simulink model "rigid_body_model"  (R2025b)
settings: Solver=ode4  StartTime=0  StopTime=10.0  FixedStep=0.001  RelTol=1e-3  EnableMultiTasking=on
undefined symbols (not defined in the file or in its folder): DiscIntNeverNeededParam
libraries: vrlib x2, aerolibutil x1
settings Model: DataDictionary=pid.sldd  EnableAccessToBaseWorkspace=off  ModifiedByFormat=The MathWorks Inc.  Creator=The MathWorks, Inc.  LastModifiedBy=The MathWorks Inc.
settings SolverCC: AlgebraicLoopSolver=TrustRegion
settings DataIOCC: ReturnWorkspaceOutputs=off
settings OptimizationCC: BlockReduction=off  DefaultParameterBehavior=Inlined  InlineInvariantSignals=on  BufferReuse=off  PassReuseOutputArgsAs=Individual arguments  ExpressionDepthLimit=2147483647.0  ZeroExternalMemoryAtStartup=off  ZeroInternalMemoryAtStartup=off  EfficientFloat2IntCast=on  LifeSpan=1  EfficientTunableParamExpr=on
settings DebuggingCC: AlgebraicLoopMsg=none  FcnCallInpInsideContextMsg=warning  UniqueDataStoreMsg=error  AssertControl=DisableAll  AllowSymbolicDim=off  StateNameClashWarn=warning  StrictBusMsg=ErrorOnBusTreatedAsVector  SFUnexpectedBacktrackingDiag=warning  SFNoUnconditionalDefaultTransitionDiag=warning  SFExecutionAtInitializationDiag=none  ArithmeticOperatorsInVariantConditions=warning
settings HardwareCC: ProdBitPerPointer=32.0  ProdBitPerSizeT=32.0  ProdBitPerPtrDiffT=32.0  ProdLargestAtomicFloat=None  ProdIntDivRoundTo=Undefined  ProdEndianess=Unspecified  ProdWordSize=32.0  ProdHWDeviceType=32-bit Generic
settings ModelReferenceCC: EnableRefExpFcnMdlSchedulingChecks=on  PropagateSignalLabelsOutOfModel=off
settings SFSimCC: SimUseLocalCustomCode=off  CustomCodeUndefinedFunction=UseInterfaceOnly
settings RTWCC: SystemTargetFile=ert.tlc  TemplateMakefile=ert_default_tmf  GenerateReport=on  RTWUseLocalCustomCode=off  IncludeHyperlinkInReport=on  GenerateTraceInfo=on  GenerateTraceReport=on  GenerateTraceReportSl=on  GenerateTraceReportSf=on  GenerateTraceReportEml=on  GenerateCodeMetricsReport=on  GPUComputeCapability=3.5  DLArmComputeVersion=19.05  Description=Embedded Coder
settings CodeAppCC: IgnoreCustomStorageClasses=off  IgnoreTestpoints=on  CustomSymbolStrType=$N$R$M  StateflowObjectComments=on  InternalIdentifier=Classic
settings ERTTargetCC: ERTCustomFileTemplate=example_file_process.tlc  ConvertIfToSwitch=off  SuppressUnreachableDefaultCases=off  DynamicArrayContainerType=coder::array  MultiwordLength=2048.0  GenerateSampleERTMain=on  SupportNonFinite=off  ParenthesesLevel=Maximum
settings ConfigComp: CovMetricSettings=dw  CovSaveCumulativeToWorkspaceVar=on  CovSaveSingleToWorkspaceVar=on  CovExternalEMLEnable=off  CovSFcnEnable=off

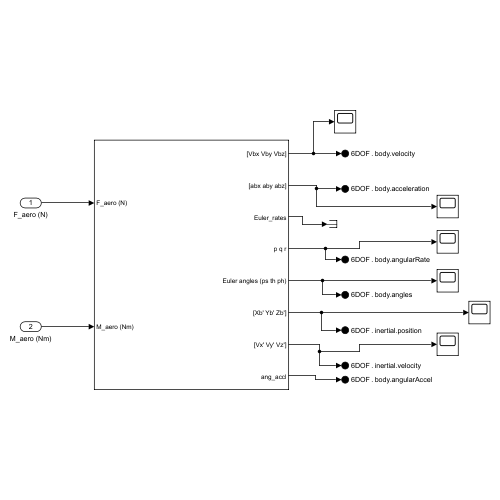
[thumbnail: Simulink's stored preview of the top-level diagram]
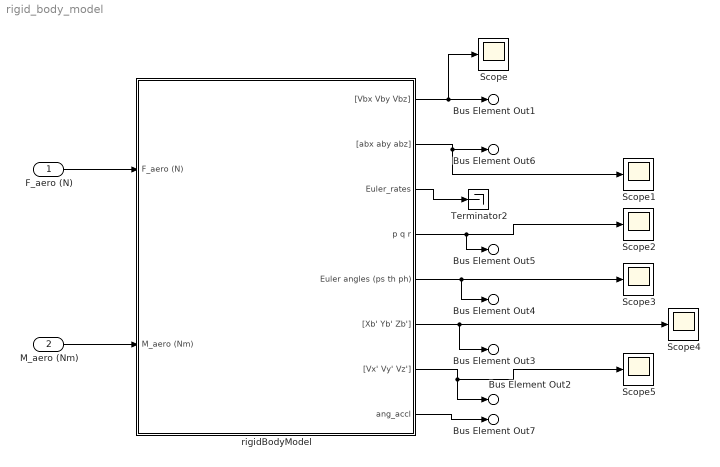
== system rigid_body_model ==
  F_aero (N) : Inport  PortDimensions=3
  M_aero (Nm) : Inport  Port=2  PortDimensions=3
  Scope{,1..5} (6 alike) : Scope
      Scope settings: ActiveDisplayYMinimum=-3.3667697972665165  ActiveDisplayYMaximum=3.6462998602310797
      Scope1 settings: ActiveDisplayYMinimum=-5.0415104437648826E+60  ActiveDisplayYMaximum=4.79275711289561E+60  DataLoggingVariableName=ScopeData2
      Scope2 settings: ActiveDisplayYMinimum=-3.6964469168621719  ActiveDisplayYMaximum=4.3336377029010054  DataLoggingVariableName=ScopeData3
      Scope3 settings: ActiveDisplayYMinimum=-0.15051515492555492  ActiveDisplayYMaximum=0.20760201896329444  DataLoggingVariableName=ScopeData4
      Scope4 settings: ActiveDisplayYMinimum=-0.00018500944845913292  ActiveDisplayYMaximum=0.0013947118751504368  DataLoggingVariableName=ScopeData5
      Scope5 settings: ActiveDisplayYMinimum=-74.102476128449538  ActiveDisplayYMaximum=562.81355446598127  DataLoggingVariableName=ScopeData6
  Terminator2 : Terminator
  rigidBodyModel : Subsystem
  Bus Element Out1 : Outport  PortName=6DOF  Element=body.velocity
  Bus Element Out4 : Outport  PortName=6DOF  Element=body.angles
  Bus Element Out6 : Outport  PortName=6DOF  Element=body.acceleration
  Bus Element Out5 : Outport  PortName=6DOF  Element=body.angularRate
  Bus Element Out7 : Outport  PortName=6DOF  Element=body.angularAccel
  Bus Element Out2 : Outport  PortName=6DOF  Element=inertial.velocity
  Bus Element Out3 : Outport  PortName=6DOF  Element=inertial.position
  wires:
  rigidBodyModel/1("[Vbx Vby Vbz]") -> Scope/1, Bus Element Out1/1
  rigidBodyModel/2("[abx aby abz]") -> Scope1/1, Bus Element Out6/1
  rigidBodyModel/3(Euler_rates) -> Terminator2/1
  rigidBodyModel/5(Euler angles (ps th ph)) -> Scope3/1, Bus Element Out4/1
  rigidBodyModel/4(p q r) -> Scope2/1, Bus Element Out5/1
  rigidBodyModel/7("[Vx' Vy' Vz']") -> Bus Element Out2/1, Scope5/1
  rigidBodyModel/6("[Xb' Yb' Zb']") -> Bus Element Out3/1, Scope4/1
  rigidBodyModel/8(ang_accl) -> Bus Element Out7/1
  M_aero (Nm)/1 -> rigidBodyModel/2(M_aero (Nm))
  F_aero (N)/1 -> rigidBodyModel/1(F_aero (N))

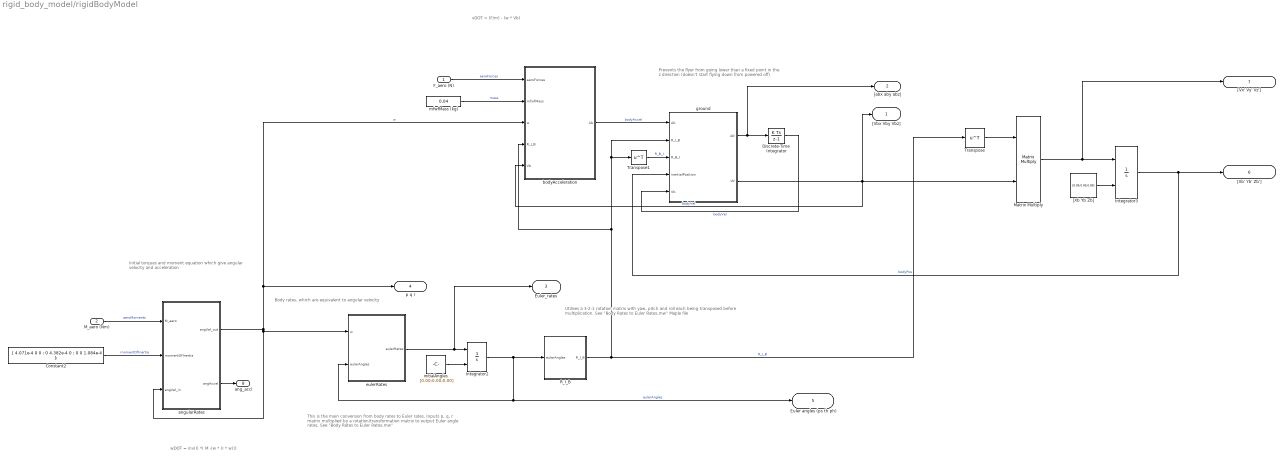
== system rigid_body_model/rigidBodyModel ==
  note: Utilises a 3-2-1 rotation matrix with yaw, pitch and roll each being transposed before multiplication. See "Body Rates to Euler Rates.mw" Maple file
  note: Prevents the flyer from going lower than a fixed point
      | in the z direction (doesn't start flying down from powered
      | off)
  note: Body rates, which are equivalent to angular velocity
  note: This is the main conversion from body rates to Euler rates.
      | Inputs p, q, r matrix multiplied by a rotation/transformation
      | matrix to output Euler angle rates. See "Body Rates to Euler Rates.mw"
  note: Initial torques and moment equation which give angular
      | velocity and acceleration
  note: wDOT = inv(I) *( M -(w * (I * w)))
  note: vDOT = (F/m) - (w * Vb)
  F_aero (N) : Inport
  M_aero (Nm) : Inport  Port=2
  Constant2 : Constant  Value=[ 4.071e-4 0 0 ; 0 4.382e-4 0 ; 0 0 1.084e-4 ];
  Discrete-Time Integrator : DiscreteIntegrator  SampleTime=-1  ICPrevOutput=DiscIntNeverNeededParam  ICPrevScaledInput=DiscIntNeverNeededParam
  Integrator2 : Integrator  InitialConditionSource=external
  Integrator3 : Integrator  InitialConditionSource=external  ShowStatePort=on
  Matrix Multiply : Product  Multiplication=Matrix(*)
  R_I_B : Subsystem
      mask Display: disp('R_I_B');
  Transpose : Math  Operator=transpose
  Transpose1 : Math  Operator=transpose
  "[Xb Yb Zb]" : Constant  Value=[0.00;0.00;0.00]
  angularRates : Subsystem
      mask Display: disp('Angular Rates');
  bodyAcceleration : Subsystem
      mask Display: disp('Body Acceleration');
  eulerRates : Subsystem
      mask Display: disp('Euler Rates');
  ground : Subsystem
      mask Display: disp('Ground');
  initialAngles : Constant  Value=[0.00;0.00;0.00]
  mfwfMass (kg) : Constant  Value=0.04
  "[Vbx Vby Vbz]" : Outport
  "[abx aby abz]" : Outport  Port=2
  Euler_rates : Outport  Port=3
  p q r : Outport  Port=4
  Euler angles (ps th ph) : Outport  Port=5
  "[Xb' Yb' Zb']" : Outport  Port=6
  "[Vx' Vy' Vz']" : Outport  Port=7
  ang_accl : Outport  Port=8
  wires:
  initialAngles/1 -> Integrator2/2
  M_aero (Nm)/1 -> angularRates/1(M_aero)  "aeroMoments"
  eulerRates/1(eulerRates) -> Integrator2/1, Euler_rates/1
  Transpose/1 -> Matrix Multiply/1
  "[Xb Yb Zb]"/1 -> Integrator3/2
  angularRates/1(angVel_out) -> angularRates/3(angVel_in), eulerRates/1(w), p q r/1, bodyAcceleration/3(w)  "w"
  Constant2/1 -> angularRates/2(momentOfInertia)  "momentOfInertia"
  Matrix Multiply/1 -> "[Vx' Vy' Vz']"/1, Integrator3/1
  ground/2(vb') -> "[Vbx Vby Vbz]"/1, Matrix Multiply/2, bodyAcceleration/5(Vb)  "bodyVel"
  Integrator3/1 -> "[Xb' Yb' Zb']"/1, ground/4(inertialPosition)  "bodyPos"
  Integrator2/1 -> Euler angles (ps th ph)/1, eulerRates/2(eulerAngles), R_I_B/1(eulerAngles)  "eulerAngles"
  R_I_B/1(R_I_B) -> bodyAcceleration/4(R_I_B), Transpose1/1, ground/2(R_I_B), Transpose/1  "R_I_B"
  angularRates/2(angAccel) -> ang_accl/1
  ground/1(Ab') -> "[abx aby abz]"/1, Discrete-Time Integrator/1
  Discrete-Time Integrator/1 -> ground/5(Vb)  "bodyVel"
  mfwfMass (kg)/1 -> bodyAcceleration/2(mfwfMass)  "mass"
  bodyAcceleration/1(Ab) -> ground/1(Ab)  "bodyAccel"
  Transpose1/1 -> ground/3(R_B_I)  "R_B_I"
  F_aero (N)/1 -> bodyAcceleration/1(aeroForces)  "aeroForces"

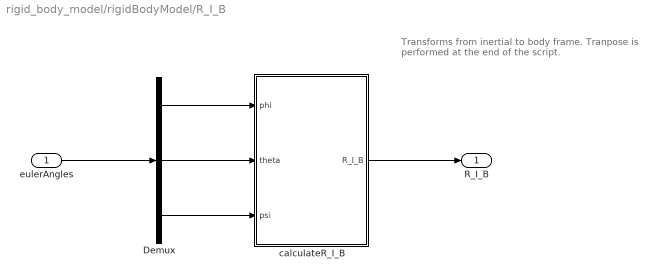
== system rigid_body_model/rigidBodyModel/R_I_B ==
  note: Transforms from inertial to body frame. Tranpose is
      | performed at the end of the script.
  eulerAngles : Inport
  Demux : Demux  Outputs=[1;1;1]
  calculateR_I_B : MATLAB Function  TreatAsAtomicUnit=on
  R_I_B : Outport
  wires:
  eulerAngles/1 -> Demux/1
  Demux/2 -> calculateR_I_B/2(theta)
  calculateR_I_B/1(R_I_B) -> R_I_B/1
  Demux/1 -> calculateR_I_B/1(phi)
  Demux/3 -> calculateR_I_B/3(psi)

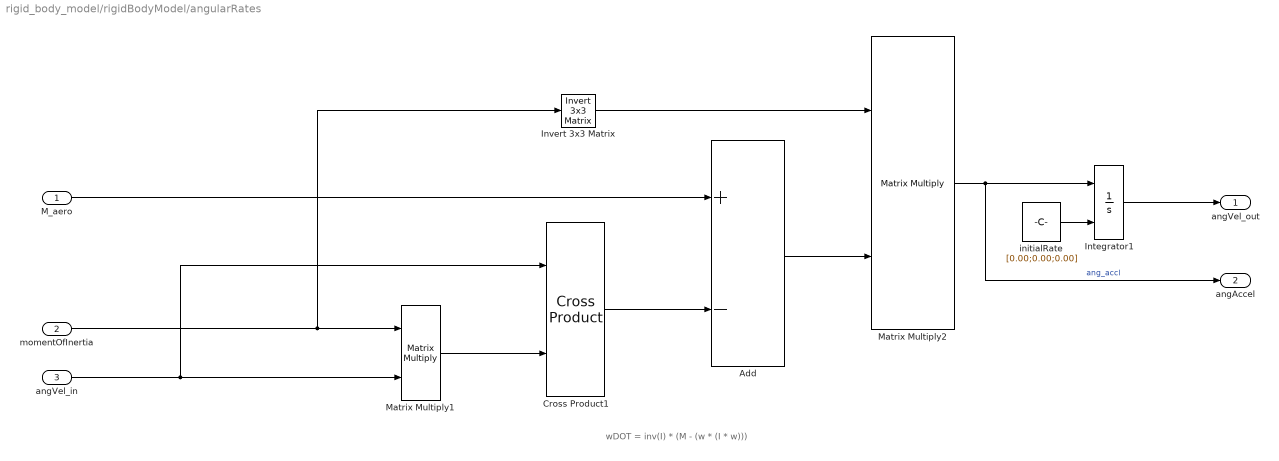
== system rigid_body_model/rigidBodyModel/angularRates ==
  note: wDOT = inv(I) * (M - (w * (I * w)))
  M_aero : Inport
  momentOfInertia : Inport  Port=2
  angVel_in : Inport  Port=3
  Add : Sum  Inputs=+-
  Cross Product1 : vrlib/Utilities/Cross Product
  Integrator1 : Integrator  InitialConditionSource=external
  Invert 3x3 Matrix : aerolibutil/Invert  3x3 Matrix
  Matrix Multiply1 : Product  Multiplication=Matrix(*)
  Matrix Multiply2 : Product  Multiplication=Matrix(*)
  initialRate : Constant  Value=[0.00;0.00;0.00]
  angVel_out : Outport
  angAccel : Outport  Port=2
  wires:
  momentOfInertia/1 -> Invert 3x3 Matrix/1, Matrix Multiply1/1
  angVel_in/1 -> Cross Product1/1, Matrix Multiply1/2
  Matrix Multiply1/1 -> Cross Product1/2
  Cross Product1/1 -> Add/2
  M_aero/1 -> Add/1
  Invert 3x3 Matrix/1 -> Matrix Multiply2/1
  Matrix Multiply2/1 -> Integrator1/1, angAccel/1  "ang_accl"
  initialRate/1 -> Integrator1/2
  Integrator1/1 -> angVel_out/1
  Add/1 -> Matrix Multiply2/2

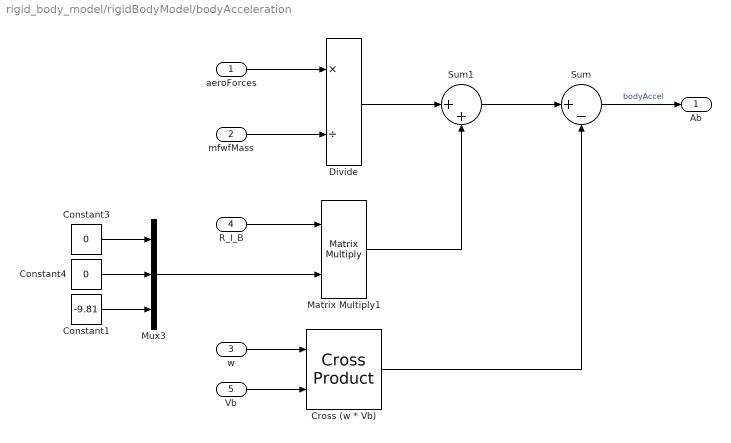
== system rigid_body_model/rigidBodyModel/bodyAcceleration ==
  aeroForces : Inport
  mfwfMass : Inport  Port=2
  w : Inport  Port=3
  R_I_B : Inport  Port=4
  Vb : Inport  Port=5
  Constant1 : Constant  Value=-9.81
  Constant3 : Constant  Value=0
  Constant4 : Constant  Value=0
  Cross (w * Vb) : vrlib/Utilities/Cross Product
  Divide : Product  Inputs=*/
  Matrix Multiply1 : Product  Multiplication=Matrix(*)
  Mux3 : Mux  Inputs=3
  Sum : Sum  Inputs=|+-
  Sum1 : Sum  Inputs=|++
  Ab : Outport
  wires:
  mfwfMass/1 -> Divide/2
  Mux3/1 -> Matrix Multiply1/2
  Divide/1 -> Sum1/1
  Matrix Multiply1/1 -> Sum1/2
  Sum1/1 -> Sum/1
  Constant3/1 -> Mux3/1
  Constant4/1 -> Mux3/2
  Constant1/1 -> Mux3/3
  R_I_B/1 -> Matrix Multiply1/1
  Sum/1 -> Ab/1  "bodyAccel"
  aeroForces/1 -> Divide/1
  w/1 -> Cross (w * Vb)/1
  Vb/1 -> Cross (w * Vb)/2
  Cross (w * Vb)/1 -> Sum/2

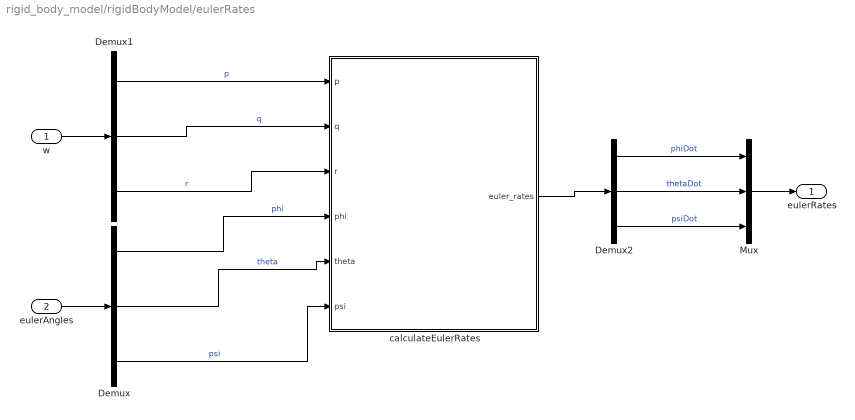
== system rigid_body_model/rigidBodyModel/eulerRates ==
  w : Inport
  eulerAngles : Inport  Port=2
  Demux : Demux  Outputs=[-1;1;1]
  Demux1 : Demux  Outputs=[1;1;1]
  Demux2 : Demux  Outputs=3
  Mux : Mux  Inputs=3
  calculateEulerRates : MATLAB Function  TreatAsAtomicUnit=on
  eulerRates : Outport
  wires:
  eulerAngles/1 -> Demux/1
  w/1 -> Demux1/1
  Demux1/2 -> calculateEulerRates/2(q)  "q"
  Demux1/1 -> calculateEulerRates/1(p)  "p"
  Demux1/3 -> calculateEulerRates/3(r)  "r"
  calculateEulerRates/1(euler_rates) -> Demux2/1
  Demux2/2 -> Mux/2  "thetaDot"
  Demux2/1 -> Mux/1  "phiDot"
  Demux2/3 -> Mux/3  "psiDot"
  Mux/1 -> eulerRates/1
  Demux/2 -> calculateEulerRates/5(theta)  "theta"
  Demux/1 -> calculateEulerRates/4(phi)  "phi"
  Demux/3 -> calculateEulerRates/6(psi)  "psi"

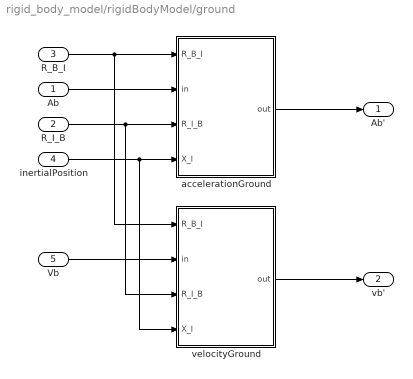
== system rigid_body_model/rigidBodyModel/ground ==
  Ab : Inport
  R_I_B : Inport  Port=2
  R_B_I : Inport  Port=3
  inertialPosition : Inport  Port=4
  Vb : Inport  Port=5
  accelerationGround : Subsystem
      mask Display: disp('Acceleration');
  velocityGround : Subsystem
      mask Display: disp('Velocity');
  Ab' : Outport
  vb' : Outport  Port=2
  wires:
  velocityGround/1(out) -> vb'/1
  R_B_I/1 -> accelerationGround/1(R_B_I), velocityGround/1(R_B_I)
  Vb/1 -> velocityGround/2(in)
  accelerationGround/1(out) -> Ab'/1
  Ab/1 -> accelerationGround/2(in)
  inertialPosition/1 -> accelerationGround/4(X_I), velocityGround/4(X_I)
  R_I_B/1 -> accelerationGround/3(R_I_B), velocityGround/3(R_I_B)

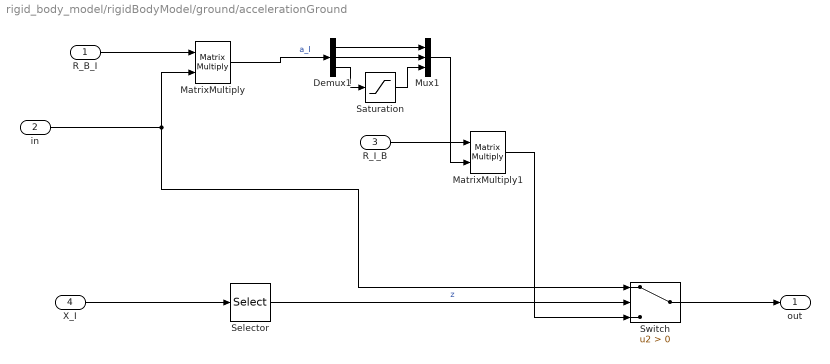
== system rigid_body_model/rigidBodyModel/ground/accelerationGround ==
  R_B_I : Inport
  in : Inport  Port=2
  R_I_B : Inport  Port=3
  X_I : Inport  Port=4
  Demux1 : Demux  Outputs=3
  MatrixMultiply : Product  Multiplication=Matrix(*)
  MatrixMultiply1 : Product  Multiplication=Matrix(*)
  Mux1 : Mux  Inputs=3
  Saturation : Saturate  UpperLimit=inf  LowerLimit=0
  Selector : Selector  InputPortWidth=3  IndexOptions=Index vector (dialog)  Indices=[3]  OutputSizes=1
  Switch : Switch  Criteria=u2 > Threshold  SaturateOnIntegerOverflow=off  InputSameDT=off
  out : Outport
  wires:
  Mux1/1 -> MatrixMultiply1/2
  Demux1/3 -> Saturation/1
  in/1 -> MatrixMultiply/2, Switch/1
  Saturation/1 -> Mux1/3
  MatrixMultiply1/1 -> Switch/3
  Selector/1 -> Switch/2  "z"
  MatrixMultiply/1 -> Demux1/1  "a_I"
  Demux1/2 -> Mux1/2
  Demux1/1 -> Mux1/1
  R_I_B/1 -> MatrixMultiply1/1
  X_I/1 -> Selector/1
  R_B_I/1 -> MatrixMultiply/1
  Switch/1 -> out/1

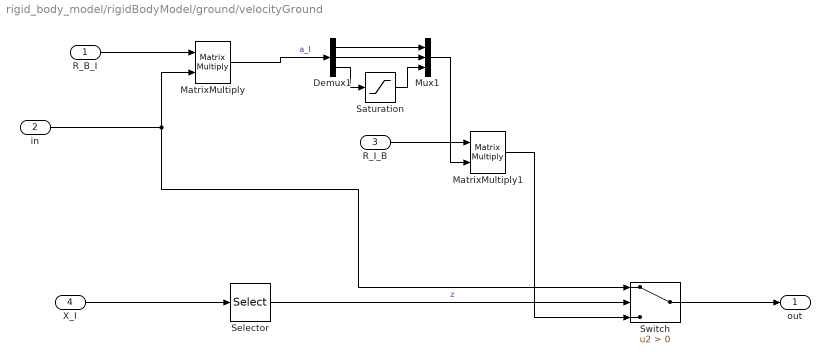
== system rigid_body_model/rigidBodyModel/ground/velocityGround ==
  R_B_I : Inport
  in : Inport  Port=2
  R_I_B : Inport  Port=3
  X_I : Inport  Port=4
  Demux1 : Demux  Outputs=3
  MatrixMultiply : Product  Multiplication=Matrix(*)
  MatrixMultiply1 : Product  Multiplication=Matrix(*)
  Mux1 : Mux  Inputs=3
  Saturation : Saturate  UpperLimit=inf  LowerLimit=0
  Selector : Selector  InputPortWidth=3  IndexOptions=Index vector (dialog)  Indices=[3]  OutputSizes=1
  Switch : Switch  Criteria=u2 > Threshold  SaturateOnIntegerOverflow=off  InputSameDT=off
  out : Outport
  wires:
  Mux1/1 -> MatrixMultiply1/2
  Demux1/3 -> Saturation/1
  in/1 -> MatrixMultiply/2, Switch/1
  Saturation/1 -> Mux1/3
  MatrixMultiply1/1 -> Switch/3
  Selector/1 -> Switch/2  "z"
  MatrixMultiply/1 -> Demux1/1  "a_I"
  Demux1/2 -> Mux1/2
  Demux1/1 -> Mux1/1
  R_I_B/1 -> MatrixMultiply1/1
  X_I/1 -> Selector/1
  R_B_I/1 -> MatrixMultiply/1
  Switch/1 -> out/1

== matlab function rigid_body_model/rigidBodyModel/eulerRates/calculateEulerRates ==
  data: p input; q input; r input; phi input; theta input; psi input; euler_rates output
function euler_rates = eulerRates(p,q,r,phi,theta, psi) 
%These equations are based of the derivation for euler rates by Colin. The
%derivation can be found inside the MS Teams.
%
%This function inputs angles and angular rates, and outputs euler rates

% This can be found in Body Rates to Euler Rates Derivation.mw, Eq 18

  euler_rates = [ p + tan(theta)*sin(phi)*q + tan(theta)*cos(phi)*r  ;
                 cos(phi)*q - sin(phi)*r                            ;
                 sin(phi)*q/cos(theta) + cos(phi)*r/cos(theta)      ;
               ];

% euler_rates = [ p + tan(theta)*sin(psi)*q + tan(theta)*cos(psi)*r  ;
%                  cos(psi)*q - sin(psi)*r                            ;
%                  sin(psi)*q/cos(theta) + cos(psi)*r/cos(theta)      ;
%                ];           
end

== matlab function rigid_body_model/rigidBodyModel/R_I_B/calculateR_I_B ==
  data: phi input; theta input; psi input; R_I_B output
function R_I_B = calc_R_I_B(phi, theta, psi)

%This function simply creates a rotation matrix from the intertial frame to 
% the body frame

% This can be found in Body Rates to Euler Rates Derivation.mw, Eq 7 (SO3
% matrix)

%Rotation from the body frame to intertial frame
R_B_I = [                 cos(theta)*cos(psi)      sin(phi)*sin(theta)*cos(psi)+cos(phi)*sin(psi)      -cos(phi)*sin(theta)*cos(psi)+sin(phi)*sin(psi)
                         -cos(theta)*sin(psi)     -sin(phi)*sin(theta)*sin(psi)+cos(phi)*cos(psi)       cos(phi)*sin(theta)*sin(psi)+sin(phi)*cos(psi)
                               sin(theta)                       -sin(phi)*cos(theta)                                cos(phi)*cos(theta)  
        ];

% taking the transpose to get the roation matrix from intertial to body frame    
R_I_B = R_B_I.'; 
end
% R_B_I = [                 cos(theta)*cos(psi)      sin(phi)*sin(theta)*cos(psi)-cos(phi)*sin(psi)      cos(phi)*sin(theta)*cos(psi)+sin(phi)*sin(psi)
%                          cos(theta)*sin(psi)     sin(phi)*sin(theta)*sin(psi)+cos(phi)*cos(psi)       cos(phi)*sin(theta)*sin(psi)-sin(phi)*cos(psi)
%                                -sin(theta)                       sin(phi)*cos(theta)                                cos(phi)*cos(theta)  
%         ];
% 
% R_I_B = R_B_I.';
